simulink model "sldrtex_filter01"  (R2015a)
settings: Solver=ode5  StartTime=0.0  StopTime=10.0  RelTol=1e-3
PostLoadFcn:
  | if ~exist('dsparch4','file') sldrtexcb_delayederror(gcs, 'Missing Library', 'This model requires DSP System Toolbox.'); end
libraries: dsparch4 x1
Description:
  | Real-Time Filter
  | 
  | This model shows a real-time filter built using DSP System Toolbox(TM) and Simulink
  | Desktop Real-Time(TM). The unfiltered signal is acquired by the analog input, passed
  | through a filter designed by DSP System Toolbox and finally sent to analog output.
  | Both the unfiltered and filtered signals are shown in real-time using the Scope block.
  | 
  | How to run this model in Normal Mode:
  | 
  | 1) Open the Analog Input and Analog Output blocks and select your data acquisition
  |    board. If there's no board installed, install it using the Install new board button.
  | 2) Double-click the orange button to switch to Normal Mode if needed.
  | 3) Start the real-time execution using Simulation->Run.
  | 
  | How to run this model in External Mode:
  | 
  | 1) Open the Analog Input and Analog Output blocks and select your data acquisition
  |    board. If there's no board installed, install it using the Install new board button.
  | 2) Double-click the orange button to switch to External Mode if needed.
  | 3) Start the real-time execution using Simulation->Run. The model will automatically
  |   build, connect to Simulink in External Mode and start.
  | 
  | Note:
  |  To run this model, you must have a data acquisition board connected to your
  |   computer.
  |  This model requires DSP System Toolbox.
settings Model: CovSFcnEnable=off  ExtModeTrigType=signal  Creator=The MathWorks Inc.  LastModifiedBy=liuqi
settings DataIOCC: SignalLoggingName=logsOut
settings OptimizationCC: ExpressionDepthLimit=2147483647  InitFltsAndDblsToZero=on  EfficientMapNaN2IntZero=off
settings DebuggingCC: UnderspecifiedInitializationDetection=Classic  MergeDetectMultiDrivingBlocksExec=none  SignalResolutionControl=TryResolveAllWithWarning  FcnCallInpInsideContextMsg=UseLocalSettings  StateNameClashWarn=warning
settings HardwareCC: ProdBitPerLong=64  ProdBitPerPointer=64  ProdIntDivRoundTo=Zero  ProdEndianess=LittleEndian  ProdWordSize=64  ProdHWDeviceType=Intel->x86-64  TargetBitPerLong=64  TargetBitPerPointer=64  TargetIntDivRoundTo=Zero  TargetEndianess=LittleEndian  TargetWordSize=64  TargetHWDeviceType=Intel->x86-64
settings RTWCC: SystemTargetFile=rtwin.tlc  TemplateMakefile=rtwin.tmf  Description=Simulink Desktop Real-Time
settings RTWinTargetCC: TargetPreCompLibLocation=F:\Program Files\MATLAB\MATLAB Production Server\R2015a\toolbox\sldrt\lib\win64

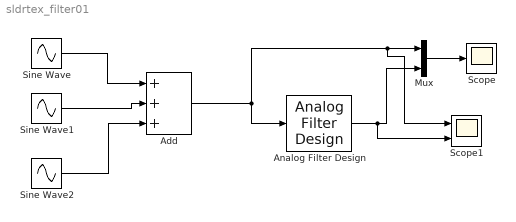
== system sldrtex_filter01 ==
  Add : Sum  Inputs=+++
  Analog Filter Design : dsparch4/Analog Filter Design  method=Butterworth  filttype=Lowpass  N=21  Wlo=12  Whi=80  Rp=3  Rs=40
  Mux : Mux  Inputs=2
  Scope : Scope
      settings: TimeRange=0.2  YMin=-1.25659  YMax=1.28483  DataFormat=Structure
  Scope1 : Scope  NumInputPorts=2
      settings: TimeRange=0.2  YMin=-1.25659~-5  YMax=1.28483~5  DataFormat=Structure
  Sine Wave : Sin  Amplitude=10  Frequency=7  SampleTime=0
  Sine Wave1 : Sin  Amplitude=5  Frequency=20  SampleTime=0
  Sine Wave2 : Sin  Amplitude=2  Frequency=35  SampleTime=0
  wires:
  Mux/1 -> Scope/1
  Analog Filter Design/1 -> Scope1/2, Mux/2
  Add/1 -> Analog Filter Design/1, Scope1/1, Mux/1
  Sine Wave/1 -> Add/1
  Sine Wave1/1 -> Add/2
  Sine Wave2/1 -> Add/3
